simulink model "DDWMR"  (R2022a)
settings: Solver=FixedStepAuto  StartTime=0.0  StopTime=T_final  FixedStep=1e-3  MaxStep=1e-2  RelTol=1e-3
values from neighbouring files (symbols this model uses):
  A1 = inv(S1)*IO*U_i.'    [Run_this_file_for_DDWMR_model.m]    (also in run_model.m; run_model_for_perform_vs_num_attack.m)
  A2 = OI*U_i.'    [Run_this_file_for_DDWMR_model.m]    (also in run_model.m; run_model_for_perform_vs_num_attack.m)
  b1p = inv(S1)*IO*U_history.'    [Run_this_file_for_DDWMR_model.m]    (also in run_model.m; run_model_for_perform_vs_num_attack.m)
  b2p = OI*U_history.'    [Run_this_file_for_DDWMR_model.m]    (also in run_model.m; run_model_for_perform_vs_num_attack.m)
  BDD_thresh = 0.1    [Run_this_file_for_DDWMR_model.m]    (also in plot_perform_vs_num_attacks.m = 0.03176; run_model.m = 0.03176)
  d = 0.1    [Run_this_file_for_DDWMR_model.m]
  e_ini_matrix = reshape(e_ini,n_meas,T1)    [Run_this_file_for_DDWMR_model.m]    (also in run_model.m; run_model_for_perform_vs_num_attack.m)
  I = Ic +mc*d^2+2*mw*L^2+2*Im    (= 0.26903125)    [Run_this_file_for_DDWMR_model.m]    (also in run_model.m = [1;2;9;11;12;16;17]; run_model_for_perform_vs_num_attack.m = sort(randperm(n_meas,n_attack)).'; test_different_horizon_size.m = sort(randperm(n_meas,n_attack)).')
  I_attack_ini = repmat(I_single,1,T1)    [Run_this_file_for_DDWMR_model.m]    (also in run_model.m = repmat(I,1,T1); run_model_for_perform_vs_num_attack.m = repmat(I,1,T1))
  I_single = sort(randperm(n_meas,n_attack)).'    [Run_this_file_for_DDWMR_model.m]
  L = 0.235/2    (= 0.1175)    [Run_this_file_for_DDWMR_model.m]    (also in encoder.m)
  m = 10    [MHFDIA_Basics.m]    (also in Run_this_file_for_DDWMR_model.m = 15; run_model.m = 19)
  max_iter = 1000    [MHFDIA_Basics.m]    (also in Perform_vs_iter.m = Max_iter(idx); Run_this_file_for_DDWMR_model.m = 2000; run_model.m = 2000; run_model_for_perform_vs_num_attack.m = 300)
  n_meas = 6    [Run_this_file_for_DDWMR_model.m]    (also in run_model.m = 19; test_different_horizon_size.m = 19)
  q_initial = [theta0;x0;y0]    [Run_this_file_for_DDWMR_model.m]
  r = 0.05    [Run_this_file_for_DDWMR_model.m]    (also in encoder.m; plot_for_different_horizon_size.m = data{1,3})
  R = 1e-3    (= 0.001)    [Run_this_file_for_DDWMR_model.m]
  T1 = 2*T    (= 12)    [Run_this_file_for_DDWMR_model.m]    (also in plot_perform_vs_num_attacks.m = 20; run_model.m = 20; test_different_horizon_size.m = T1_array(iter))
  T_start_attack = .2*T_final    (= 4)    [Run_this_file_for_DDWMR_model.m]    (also in plot_results.m = .2*T_final; run_model.m = 1.6)
  Ts = 0.01    [Run_this_file_for_DDWMR_model.m]    (also in plot_results.m)
  V_initial = [v0;omega0]    [Run_this_file_for_DDWMR_model.m]
libraries: simulink x2, sharedTrackingLibrary x1
settings Model: Creator=yz19b  LastModifiedBy=Abely
settings SolverCC: AlgebraicLoopSolver=TrustRegion
settings DebuggingCC: UnconnectedInputMsg=warning  UnconnectedOutputMsg=warning  UnconnectedLineMsg=warning  SFMachineParentedDataDiag=warning

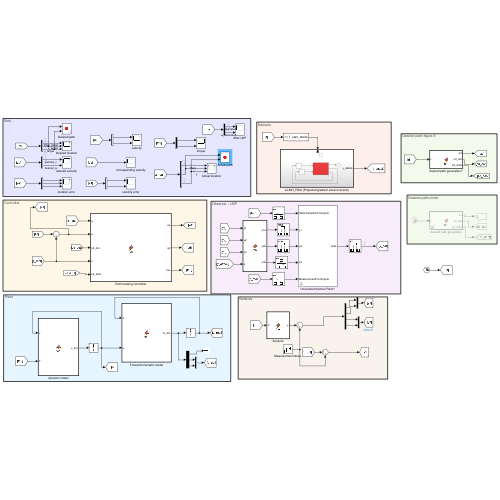
[thumbnail: Simulink's stored preview of the top-level diagram]
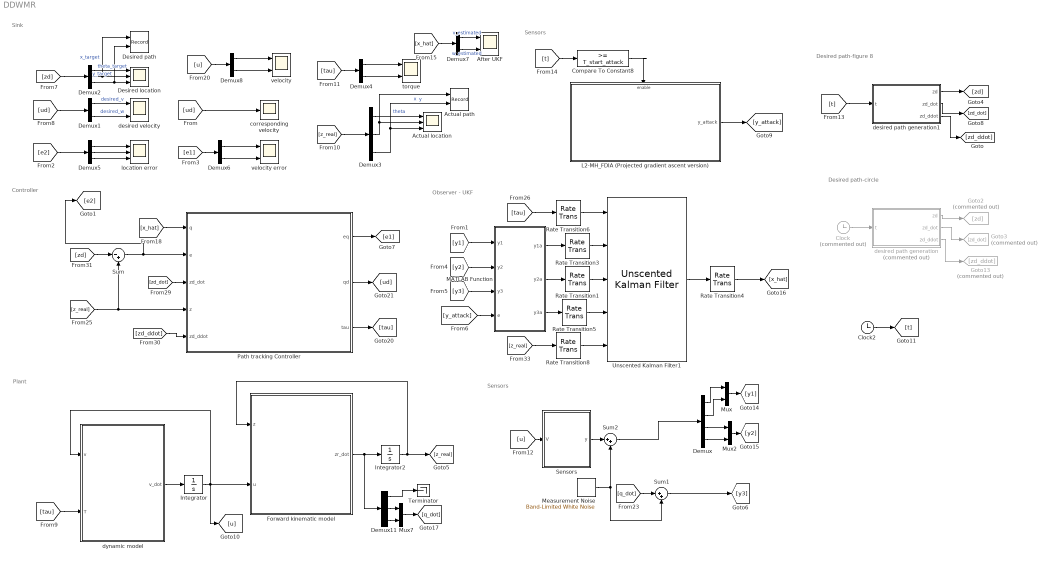
== system DDWMR ==
  note: Desired path-circle
  note: Sink
  note: Controller
  note: Plant
  note: Sensors
  note: Observer - UKF
  note: Desired path-figure 8
  note: Sensors
  Actual location : Scope  NumInputPorts=3
  Actual path : Record  FileSettingsInternal="{\"entries\":[{\"content\":{\"excelSettings\":{\"content\":{},\"type\":\"Streamout.ExcelSettings\"}},\"type\":\"Streamout.FileSettingStorage\",\"uuid\":\"92cc1c26-a867-4b51-9c3a-cf097048ddac\"}],\"packageUris\":[\"http://schema.mathworks.com/mf0/streamout_blocks/R2020a\"],\"version\":\"1.0\"}"  Layout=[1 1]  SignalsInternal="{\"entries\":[{\"content\":{\"signals\":[{\"content\":{\"blockPath\":[\"DDWMR/Actual path\"],\"channel\":[],\"dimensions\":[1],\"domain\":\"DDWMR/Actual path\",\"lineColor\":\"#a2142f\",\"plots\":[1],\"port\":1,\"sid\":[\"\"],\"signalID\":1288,\"signalName\":\"x\"},\"type\":\"RecordBlkView.Signal\",\"uuid\":\"d92e6942-c2e4-4f62-a873-64705adb8754\"},{\"content\":{\"blockPath\":[\"DDWMR/Actual path\"],\"channel\":[],\"dimensions\":[1],\"domain\":\"DDWMR/Actual path\",\"lineColor\":\"#139fff\",\"plots\":[1],\"port\":2,\"sid\":[\"\"],\"signalID\":1292,\"signalName\":\"y\"},\"type\":\"RecordBlkView.Signal\",\"uuid\":\"2719b7ca-13df-4005-bc70-abdc76224363\"}]},\"type\":\"RecordBlkView.InputSignals\",\"uuid\":\"84158e23-1399-468b-9c30-7cf538c9f3cb\"}],\"packageUris\":[\"http://schema.mathworks.com/mf0/streamout_blocks/R2020a\"],\"version\":\"1.0\"}"  VisualizationBindings="{\"xyplotplugin\":{\"info\":[{\"series\":[{\"bindingParametersList\":[{\"parameter\":\"X-Axis\",\"signalID\":1288,\"signalName\":\"x\"},{\"parameter\":\"Y-Axis\",\"signalID\":1292,\"signalName\":\"y\"}],\"seriesID\":33921}],\"subplotID\":1}]}}"  CompatibilityTag=XY  st=-1
  After UKF : Scope  NumInputPorts=2
  Clock : Clock  Commented=on
  Clock2 : Clock
  Compare To Constant8 : simulink/Logic and Bit Operations/Compare To Constant  relop=>=  const=T_start_attack  OutDataTypeStr=boolean
  Demux : Demux
  Demux{1,4,6..8} (5 alike) : Demux  Outputs=2
  Demux{2..3,5,11} (4 alike) : Demux  Outputs=3
  Desired location : Scope  NumInputPorts=3
  "Desired path " : Record  FileSettingsInternal="{\"entries\":[{\"content\":{\"excelSettings\":{\"content\":{},\"type\":\"Streamout.ExcelSettings\"}},\"type\":\"Streamout.FileSettingStorage\",\"uuid\":\"cbdf2a21-cbd5-4086-a500-666676154ed7\"}],\"packageUris\":[\"http://schema.mathworks.com/mf0/streamout_blocks/R2020a\"],\"version\":\"1.0\"}"  Layout=[1 1]  SignalsInternal="{\"entries\":[{\"content\":{\"signals\":[{\"content\":{\"blockPath\":[\"DDWMR/Desired path \"],\"channel\":[],\"dimensions\":[1],\"domain\":\"DDWMR/Desired path \",\"lineColor\":\"#a2142f\",\"plots\":[1],\"port\":1,\"sid\":[\"\"],\"signalID\":1296,\"signalName\":\"x_target\"},\"type\":\"RecordBlkView.Signal\",\"uuid\":\"e4cd04d4-903d-4b22-92da-ee0d93b25ac6\"},{\"content\":{\"blockPath\":[\"DDWMR/Desired path \"],\"channel\":[],\"dimensions\":[1],\"domain\":\"DDWMR/Desired path \",\"lineColor\":\"#139fff\",\"plots\":[1],\"port\":2,\"sid\":[\"\"],\"signalID\":1300,\"signalName\":\"y_target\"},\"type\":\"RecordBlkView.Signal\",\"uuid\":\"2bf334e2-7699-4529-b0c2-237e2c238a2b\"}]},\"type\":\"RecordBlkView.InputSignals\",\"uuid\":\"925bfc09-a75c-48b0-972f-e2951768649b\"}],\"packageUris\":[\"http://schema.mathworks.com/mf0/streamout_blocks/R2020a\"],\"version\":\"1.0\"}"  VisualizationBindings="{\"xyplotplugin\":{\"info\":[{\"series\":[{\"bindingParametersList\":[{\"parameter\":\"X-Axis\",\"signalID\":1296,\"signalName\":\"x_target\"},{\"parameter\":\"Y-Axis\",\"signalID\":1300,\"signalName\":\"y_target\"}],\"seriesID\":19807}],\"subplotID\":1}]}}"  CompatibilityTag=XY  st=-1
  Forward kinematic model : MATLAB Function  TreatAsAtomicUnit=on
  Goto13 : Goto  Commented=on  GotoTag=zd_ddot
  Goto2 : Goto  Commented=on  GotoTag=zd
  Goto3 : Goto  Commented=on  GotoTag=zd_dot
  Integrator : Integrator  InitialCondition=V_initial
  Integrator2 : Integrator  InitialCondition=q_initial
  L2-MH_FDIA (Projected gradient ascent version) : Subsystem
  MATLAB Function : MATLAB Function  TreatAsAtomicUnit=on
  Measurement Noise : simulink/Sources/Band-Limited White Noise  Cov=R*Ts  Ts=Ts  seed=[23341]
  Mux : Mux  Inputs=2
  Mux2 : Mux  Inputs=2
  Mux7 : Mux  Inputs=2
  Path tracking Controller : MATLAB Function  TreatAsAtomicUnit=on
  Rate Transition{1,3,5..6} (4 alike) : RateTransition  InitialCondition=[0 0]  OutPortSampleTime=Ts
  Rate Transition4 : RateTransition  Integrity=off  InitialCondition=1.6  OutPortSampleTime=0
  Rate Transition8 : RateTransition  InitialCondition=[0 0 0]  OutPortSampleTime=Ts
  Sensors : MATLAB Function  TreatAsAtomicUnit=on
  Sum : Sum  Inputs=|-+
  Sum1 : Sum  Inputs=|++
  Sum2 : Sum  Inputs=|++
  Terminator : Terminator
  Unscented Kalman Filter1 : sharedTrackingLibrary/Unscented Kalman Filter  StateTransitionFcn=Dynamicfcn  HasAdditiveProcessNoise=Additive  ProcessNoise=diag([1 1])  HasTimeVaryingProcessNoise=off  HasStateTransitionFcnExtraArgument=1  InitialState=[0 0]  InitialStateCovariance=1e-2  Alpha=1e-2  Beta=2  Kappa=0  MeasurementFcn1=gyroscope  HasMeasurementEnablePort1=off  HasAdditiveMeasurementNoise1=Additive  MeasurementNoise1=diag([R R])  HasTimeVaryingMeasurementNoise1=off  HasMeasurementFcnExtraArgument1=0  HasMeasurementWrapping1=off  MeasurementFcn2=encoder  HasMeasurementEnablePort2=off  HasAdditiveMeasurementNoise2=Additive  MeasurementNoise2=diag([R R])  HasTimeVaryingMeasurementNoise2=off  HasMeasurementFcnExtraArgument2=0  HasMeasurementWrapping2=off  MeasurementFcn3=gps  HasMeasurementEnablePort3=off  HasAdditiveMeasurementNoise3=Additive  MeasurementNoise3=diag([R R])  HasTimeVaryingMeasurementNoise3=off  HasMeasurementFcnExtraArgument3=1  HasMeasurementWrapping3=off  MeasurementFcn4=mfcn3  HasMeasurementEnablePort4=off  HasAdditiveMeasurementNoise4=Additive  MeasurementNoise4=R  HasTimeVaryingMeasurementNoise4=off  HasMeasurementFcnExtraArgument4=0  HasMeasurementWrapping4=off  MeasurementFcn5=myMeasurementFcn  HasMeasurementEnablePort5=off  HasAdditiveMeasurementNoise5=Additive  MeasurementNoise5=1  HasTimeVaryingMeasurementNoise5=off  HasMeasurementFcnExtraArgument5=0  HasMeasurementWrapping5=off  EnableMultirate=off  StateTransitionFcnSampleTime=1  MeasurementFcn1SampleTime=1  MeasurementFcn2SampleTime=1  MeasurementFcn3SampleTime=1  MeasurementFcn4SampleTime=1  MeasurementFcn5SampleTime=1  UseCurrentEstimator=on  OutputStateCovariance=off  DataType=double  SampleTime=Ts  NumberOfMeasurements=3
      settings: SourceProductBaseCode=TF,AE,PW,CT,DR,ID,LP,NV,AR,RO,RR,UV,VE
  corresponding velocity : Scope
  desired path generation : MATLAB Function  Commented=on  TreatAsAtomicUnit=on
  desired path generation1 : MATLAB Function  TreatAsAtomicUnit=on
  desired velocity : Scope  NumInputPorts=2
  dynamic model : MATLAB Function  TreatAsAtomicUnit=on
  location error : Scope  NumInputPorts=3
  torque : Scope  NumInputPorts=2
  velocity : Scope  NumInputPorts=2
  velocity error : Scope  NumInputPorts=2
  wires:
  Clock/1 -> desired path generation/1(t)
  [ud] -> Demux1/1
  Demux1/1 -> desired velocity/1  "desired_v"
  Demux1/2 -> desired velocity/2  "desired_w"
  desired path generation/2(zd_dot) -> Goto3/1
  desired path generation/1(zd) -> Goto2/1
  [zd] -> Demux2/1
  Demux2/1 -> Desired location/1  "theta_target"
  Demux2/2 -> "Desired path "/1, Desired location/2  "x_target"
  Demux2/3 -> "Desired path "/2, Desired location/3  "y_target"
  [tau] -> dynamic model/2(T)
  Forward kinematic model/1(zr_dot) -> Demux11/1, Integrator2/1
  Integrator2/1 -> [z_real], Forward kinematic model/1(z)
  [z_real] -> Demux3/1
  Demux3/3 -> Actual path/2, Actual location/3  "y"
  Demux3/2 -> Actual path/1, Actual location/2  "x"
  Demux3/1 -> Actual location/1  "theta"
  Demux4/2 -> torque/2
  Demux4/1 -> torque/1
  [tau] -> Demux4/1
  [e2] -> Demux5/1
  Demux5/1 -> location error/1
  Demux5/2 -> location error/2
  Demux6/2 -> velocity error/2
  Demux6/1 -> velocity error/1
  [e1] -> Demux6/1
  dynamic model/1(v_dot) -> Integrator/1
  [ud] -> corresponding velocity/1
  [u] -> Sensors/1(V)
  Sensors/1(y) -> Sum2/1
  Sum1/1 -> [y3]
  Sum2/1 -> Demux/1
  Demux8/1 -> velocity/1
  Demux8/2 -> velocity/2
  [u] -> Demux8/1
  Demux/1 -> Mux/1
  Demux/2 -> Mux/2
  Demux/3 -> Mux2/1
  Demux/4 -> Mux2/2
  Mux/1 -> [y1]
  Mux2/1 -> [y2]
  [q_dot] -> Sum1/1
  Measurement Noise/1 -> Sum1/2, Sum2/2
  Demux7/1 -> After UKF/1  "v_estimated"
  Demux7/2 -> After UKF/2  "w_estimated"
  [x_hat] -> Demux7/1
  Integrator/1 -> Forward kinematic model/2(u), dynamic model/1(v), [u]
  Rate Transition4/1 -> [x_hat]
  [tau] -> Rate Transition6/1
  Unscented Kalman Filter1/1 -> Rate Transition4/1
  Rate Transition6/1 -> Unscented Kalman Filter1/1
  Demux11/2 -> Mux7/1
  Demux11/3 -> Mux7/2
  Mux7/1 -> [q_dot]
  Demux11/1 -> Terminator/1
  [z_real] -> Rate Transition8/1
  Rate Transition8/1 -> Unscented Kalman Filter1/5
  desired path generation1/1(zd) -> [zd]
  desired path generation1/2(zd_dot) -> [zd_dot]
  [t] -> desired path generation1/1(t)
  desired path generation/3(zd_ddot) -> Goto13/1
  [z_real] -> Sum/2, Path tracking Controller/4(z)
  [zd_dot] -> Path tracking Controller/3(zd_dot)
  [zd_ddot] -> Path tracking Controller/5(zd_ddot)
  [zd] -> Sum/1
  Sum/1 -> [e2], Path tracking Controller/2(e)
  Path tracking Controller/3(tau) -> [tau]
  Path tracking Controller/2(qd) -> [ud]
  desired path generation1/3(zd_ddot) -> [zd_ddot]
  Demux5/3 -> location error/3
  Path tracking Controller/1(eq) -> [e1]
  [x_hat] -> Path tracking Controller/1(q)
  L2-MH_FDIA (Projected gradient ascent version)/1(y_attack) -> [y_attack]
  [t] -> Compare To Constant8/1
  Compare To Constant8/1 -> L2-MH_FDIA (Projected gradient ascent version)/Enable
  [y2] -> MATLAB Function/2(y2)
  [y1] -> MATLAB Function/1(y1)
  [y3] -> MATLAB Function/3(y3)
  [y_attack] -> MATLAB Function/4(e)
  MATLAB Function/1(y1a) -> Rate Transition3/1
  MATLAB Function/2(y2a) -> Rate Transition1/1
  MATLAB Function/3(y3a) -> Rate Transition5/1
  Clock2/1 -> [t]
  Rate Transition3/1 -> Unscented Kalman Filter1/2
  Rate Transition1/1 -> Unscented Kalman Filter1/3
  Rate Transition5/1 -> Unscented Kalman Filter1/4

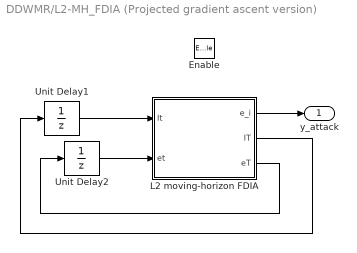
== system DDWMR/L2-MH_FDIA (Projected gradient ascent version) ==
  Enable : EnablePort
  L2 moving-horizon FDIA : MATLAB Function  TreatAsAtomicUnit=on
  Unit Delay1 : UnitDelay  InitialCondition=I_attack_ini  SampleTime=-1  HasFrameUpgradeWarning=on
  Unit Delay2 : UnitDelay  InitialCondition=e_ini_matrix  SampleTime=-1  HasFrameUpgradeWarning=on
  y_attack : Outport
  wires:
  L2 moving-horizon FDIA/1(e_i) -> y_attack/1
  Unit Delay1/1 -> L2 moving-horizon FDIA/1(It)
  Unit Delay2/1 -> L2 moving-horizon FDIA/2(et)
  L2 moving-horizon FDIA/2(IT) -> Unit Delay1/1
  L2 moving-horizon FDIA/3(eT) -> Unit Delay2/1

== matlab function DDWMR/dynamic model ==
  data: v_dot output; v input; T input; L parameter; r parameter; d parameter; m parameter; I parameter
function v_dot = fcn(v, T,L, r, d, m,I)

%% unpacking intput
omega=v(2);

%% Parameter
M_temp=[m*d*d+I,0;
         0,m];

M_inver=(1/(m*(m*d*d+I)))*M_temp;

D=[0,-m*d*omega;
    m*d*omega,0];

B=(1/r)*[1,1;L,-L];

%% ODE
v_dot=M_inver*(-D*v+B*T);

== matlab function DDWMR/desired path generation ==
  data: t input; zd output; zd_dot output; zd_ddot output
function [zd,zd_dot,zd_ddot] = fcn(t)


% unit circle (radius = 1; origin: (0,0))
zd = [t;
      cos(t);         % x
      sin(t)];        % y

zd_dot = [-sin(t);
          cos(t)];
      
zd_ddot = [-cos(t);
           -sin(t)];

== matlab function DDWMR/desired path generation1 ==
  data: t input; zd output; zd_dot output; zd_ddot output
function [zd,zd_dot,zd_ddot] = fcn(t)

a=1;
x = a*cos(t)/(1+sin(t)^2);
y = a*sin(t)*cos(t)/(1+sin(t)^2);
% unit circle (radius = 1; origin: (0,0))
zd = [atan(y./x);              % theta
      a*cos(t)/(1+sin(t)^2);         % x
      a*sin(t)*cos(t)/(1+sin(t)^2)];        % y

zd_dot = [-a*sin(t)*(cos(t)^2+2)/(1+sin(t)^2)^2;
          (a*cos(t)^2-2*a*sin(t)^2)/(1+sin(t)^2)^2];

z1 = (a*sin(t)^2*cos(t)^3-11*a*cos(t)^3+8*a*cos(t))/(1+sin(t)^2)^3;
z2 = -2*a*sin(t)*cos(t)*(3+2*cos(t)^2-sin(t)^2)/(1+sin(t)^2)^3;
zd_ddot = [z1;
           z2];

== matlab function DDWMR/L2-MH_FDIA (Projected gradient ascent version)/L2 moving-horizon FDIA ==
  data: A1 parameter; BDD_thresh parameter; It input; et input; T1 parameter; n_meas parameter; A2 parameter; b1p parameter; b2p parameter; e_i output; IT output; eT output; max_iter parameter; I_single parameter
function [e_i,IT,eT] = fcn(A1,BDD_thresh,It,et, T1, n_meas, A2, b1p, b2p,max_iter,I_single)
%% generate moving-horizon attack

%% unpacking inputs
et_temp = et(:,2:end);
e_history = et_temp;

It_temp = It(:,2:end);
I_history = It_temp;


%% solve the current attack
I_i = I_single;  % attack support

[stop_iter,e_i] = L2_MH_FDIA(A1,A2,b1p,b2p,I_history,e_history,I_i,T1,n_meas,T1*BDD_thresh,max_iter);

% eps0 = norm(A2*e_i+b2p*e_history(:));
% eps2 = norm(G2*[et(:);e_i]);
%% store the attack vectors and supports
et(:,1:end-1) = et(:,2:end);
et(:,end) = e_i;
eT = et;
% 
% eps1 = norm(G1*eT(:));


It(:,1:end-1) = It(:,2:end);
It(:,end) = I_i;
IT = It;

== matlab function DDWMR/MATLAB Function ==
  data: y1 input; y1a output; y2 input; y3 input; e input; y2a output; y3a output
function [y1a,y2a,y3a] = fcn(y1,y2,y3,e)

y1_size = length(y1);
y2_size = length(y2);
% y3_size = length(y3);

y1a = y1 + e(1:y1_size);
y2a = y2 + e(y1_size+1:y1_size+y2_size);
y3a = y3 + e(y1_size+y2_size+1:end);

== matlab function DDWMR/Sensors ==
  data: V input; y output; r parameter; L parameter
function y = fcn(V,r,L)

C=[1,0;
    0,1;
    1/(4*r),L/(4*r);
    1/(4*r),-L/(4*r)];
y=C*V;

== matlab function DDWMR/Path tracking Controller ==
  data: eq output; qd output; q input; tau output; e input; zd_dot input; z input; zd_ddot input; m parameter; d parameter; r parameter; L parameter; I parameter
function [eq,qd,tau] = fcn(q,e,zd_dot,z,zd_ddot,m, d, r, L, I)


kq =15;
ke =15;
ez = e(2:3);
% e_theta = e(1);
theta = z(1);
omega = q(2);

B_inver=-(r/(2*L))*[-L,-1;-L,1];
M=[m,0;
    0,m*d*d+I];
D=[0,-m*d*omega;
    m*d*omega,0];
C = [cos(theta), -d*sin(theta);
     sin(theta), d*cos(theta)];
C_bar_tran = [0, cos(theta), sin(theta);
              1, -d*sin(theta), d*cos(theta)];
C_inver = (1/d)*[d*cos(theta), d*sin(theta);
                 -sin(theta), cos(theta)];
C_inver_dot = (1/d)*[-d*sin(theta)*omega, d*cos(theta)*omega;
                     -cos(theta)*omega, -sin(theta)*omega];


qd = C_inver*(zd_dot-ke*ez);
qd_dot = -ke*(C_inver_dot*ez+q)+C_inver*(zd_ddot+ke*zd_dot+C*C_inver_dot*zd_dot);
u = -kq*(q-qd)+qd_dot-C_bar_tran*e;
tau = B_inver*(M*u+D*q);
eq = q-qd;

== matlab function DDWMR/Forward kinematic model ==
  data: z input; u input; zr_dot output; d parameter; r parameter
function zr_dot = fcn(z,u,d,r)

%% unpacking the state vectors
theta=z(1);

%% unpacking the intput
v=u(1);
omega=u(2);

%% ODE
theta_dot=omega;
x_dot=v*cos(theta)-d*omega*sin(theta);
y_dot=v*sin(theta)+d*omega*cos(theta);
% phir_dot = (v+omega)/r;
% phil_dot = (v-omega)/r;


%% packing the output
zr_dot=[theta_dot;x_dot;y_dot];
